simulink model "lat_noInput"  (R2016a)
settings: Solver=VariableStepAuto  StartTime=0.0  StopTime=200  RelTol=1e-3
undefined symbols (not defined in the file): Alat, Blat, Clat, Dlat
settings Model: Creator=Gray  LastModifiedBy=Gray

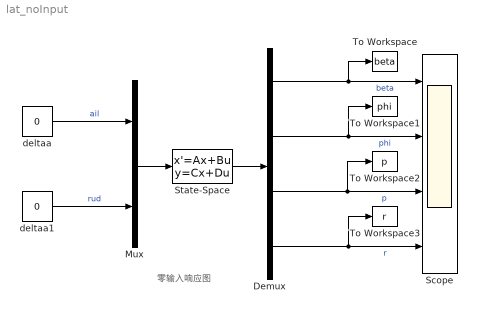
== system lat_noInput ==
  note: 零输入响应图
  Demux : Demux
  Mux : Mux  Inputs=2
  Scope : Scope  NumInputPorts=4
  State-Space : StateSpace  A=Alat  B=Blat  C=Clat  D=Dlat  X0="[5/57.3  0 0 0]'"
  To Workspace : ToWorkspace  VariableName=beta  SaveFormat=Timeseries  SampleTime=-1
  To Workspace1 : ToWorkspace  VariableName=phi  SaveFormat=Timeseries  SampleTime=-1
  To Workspace2 : ToWorkspace  VariableName=p  SaveFormat=Timeseries  SampleTime=-1
  To Workspace3 : ToWorkspace  VariableName=r  SaveFormat=Timeseries  SampleTime=-1
  deltaa : Constant  Value=0
  deltaa1 : Constant  Value=0
  wires:
  State-Space/1 -> Demux/1
  Mux/1 -> State-Space/1
  Demux/1 -> To Workspace/1, Scope/1  "beta"
  Demux/2 -> To Workspace1/1, Scope/2  "phi"
  Demux/3 -> Scope/3, To Workspace2/1  "p"
  Demux/4 -> To Workspace3/1, Scope/4  "r"
  deltaa1/1 -> Mux/2  "rud"
  deltaa/1 -> Mux/1  "ail"
